simulink model "SRP_torque"  (R2021b)
settings: Solver=VariableStepAuto  StartTime=0.0  StopTime=10.0  MaxStep=1e-2  RelTol=1e-13
values from neighbouring files (symbols this model uses):
  c = 3e8    (= 300000000)    [Lab_7.m]
  N_B = [1 0 0]    [Lab_7.m]
  rho_d = 1    [Lab_7.m]
  rho_s = 0.5    [Lab_7.m]
undefined symbols (not defined in the file or in its folder): A, r_MB, r_SP1, r_SP2, S_B
libraries: matrix_library x3
settings Model: Creator=adity  LastModifiedBy=adity

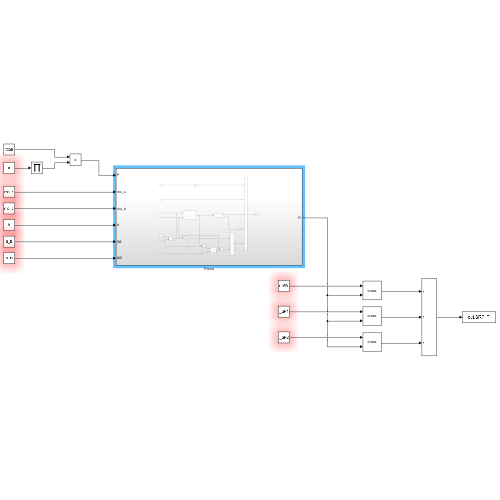
[thumbnail: Simulink's stored preview of the top-level diagram]
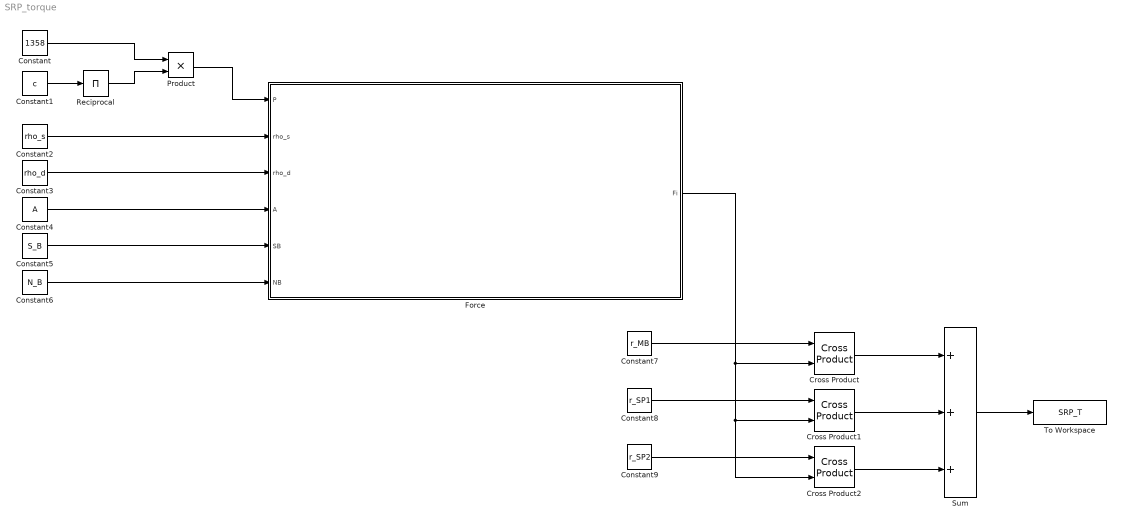
== system SRP_torque ==
  Constant : Constant  Value=1358
  Constant1 : Constant  Value=c
  Constant2 : Constant  Value=rho_s
  Constant3 : Constant  Value=rho_d
  Constant4 : Constant  Value=A
  Constant5 : Constant  Value=S_B
  Constant6 : Constant  Value=N_B
  Constant7 : Constant  Value=r_MB
  Constant8 : Constant  Value=r_SP1
  Constant9 : Constant  Value=r_SP2
  Cross Product : matrix_library/Cross Product
      settings: SourceProductBaseCode=SL
  Cross Product1 : matrix_library/Cross Product
      settings: SourceProductBaseCode=SL
  Cross Product2 : matrix_library/Cross Product
      settings: SourceProductBaseCode=SL
  Force : Subsystem
  Product : Product
  Reciprocal : Product  Inputs=1
  Sum : Sum  Inputs=+++
  To Workspace : ToWorkspace  VariableName=SRP_T  SaveFormat=Timeseries  SampleTime=-1
  wires:
  Constant1/1 -> Reciprocal/1
  Constant/1 -> Product/1
  Reciprocal/1 -> Product/2
  Product/1 -> Force/1(P)
  Constant2/1 -> Force/2(rho_s)
  Constant3/1 -> Force/3(rho_d)
  Constant4/1 -> Force/4(A)
  Constant5/1 -> Force/5(SB)
  Constant6/1 -> Force/6(NB)
  Cross Product/1 -> Sum/1
  Cross Product1/1 -> Sum/2
  Cross Product2/1 -> Sum/3
  Sum/1 -> To Workspace/1
  Constant7/1 -> Cross Product/1
  Constant8/1 -> Cross Product1/1
  Constant9/1 -> Cross Product2/1
  Force/1(Fi) -> Cross Product/2, Cross Product1/2, Cross Product2/2

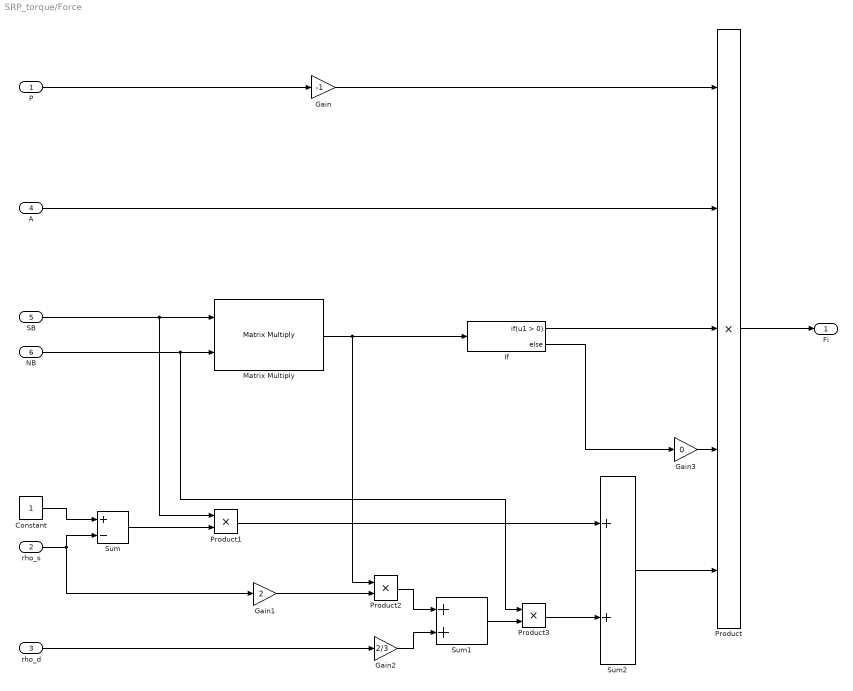
== system SRP_torque/Force ==
  P : Inport
  rho_s : Inport  Port=2
  rho_d : Inport  Port=3
  A : Inport  Port=4
  SB : Inport  Port=5
  NB : Inport  Port=6
  Constant : Constant
  Gain : Gain  Gain=-1
  Gain1 : Gain  Gain=2
  Gain2 : Gain  Gain=2/3
  Gain3 : Gain  Gain=0
  If : If
  Matrix Multiply : Product  Multiplication=Matrix(*)
  Product : Product  Inputs=5
  Product1 : Product
  Product2 : Product
  Product3 : Product
  Sum : Sum  Inputs=+-
  Sum1 : Sum
  Sum2 : Sum
  Fi : Outport
  wires:
  P/1 -> Gain/1
  SB/1 -> Product1/1, Matrix Multiply/1
  NB/1 -> Matrix Multiply/2, Product3/1
  A/1 -> Product/2
  Gain/1 -> Product/1
  Product/1 -> Fi/1
  Matrix Multiply/1 -> If/1, Product2/1
  Constant/1 -> Sum/1
  rho_s/1 -> Gain1/1, Sum/2
  Sum/1 -> Product1/2
  Gain1/1 -> Product2/2
  rho_d/1 -> Gain2/1
  Product2/1 -> Sum1/1
  Gain2/1 -> Sum1/2
  Sum1/1 -> Product3/2
  Product1/1 -> Sum2/1
  Product3/1 -> Sum2/2
  If/1 -> Product/3
  If/2 -> Gain3/1
  Sum2/1 -> Product/5
  Gain3/1 -> Product/4
